simulink model "Servo_Simulation"  (R2019b)
settings: Solver=VariableStepAuto  StartTime=0.0  StopTime=15.0  RelTol=1e-3
undefined symbols (not defined in the file): sigbuilder_block
libraries: simulink x4
settings Model: PacingRate=0.008900  Creator=michi  LastModifiedBy=michi

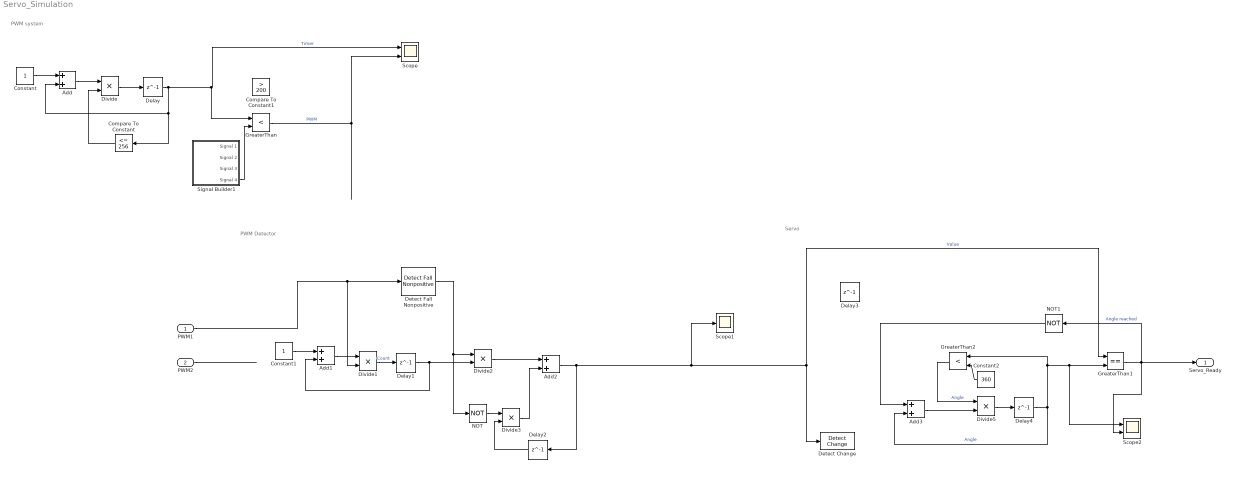
== system Servo_Simulation ==
  note: Servo
  note: PWM Detector
  note: PWM system
  PWM1 : Inport
  PWM2 : Inport  Port=2
  Add{,1..3} (4 alike) : Sum
  Compare To Constant : simulink/Logic and Bit Operations/Compare To Constant  relop=<=  const=256  OutDataTypeStr=boolean
  Compare To Constant1 : simulink/Logic and Bit Operations/Compare To Constant  relop=>  const=200  OutDataTypeStr=boolean
  Constant : Constant
  Constant1 : Constant
  Constant2 : Constant  Value=360
  Delay{,1..3} (4 alike) : Delay  DelayLength=1  SampleTime=1/12800
  Delay4 : Delay  DelayLength=1  SampleTime=0.16/60
  Detect Change : simulink/Logic and Bit Operations/Detect Change  vinit=0  OutDataTypeStr=boolean
  Detect Fall Nonpositive : simulink/Logic and Bit Operations/Detect Fall Nonpositive  vinit=1  OutDataTypeStr=boolean
      settings: SourceProductName=Simulink  SourceProductBaseCode=SL
  Divide : Product  Inputs=**  SaturateOnIntegerOverflow=on  RndMeth=Zero
  Divide1 : Product  Inputs=**  SaturateOnIntegerOverflow=on  RndMeth=Zero
  Divide2 : Product  Inputs=**
  Divide3 : Product  Inputs=**
  Divide5 : Product  Inputs=**  OutDataTypeStr=uint16  SaturateOnIntegerOverflow=on  RndMeth=Zero
  GreaterThan : RelationalOperator  Operator=<  OutDataTypeStr=boolean  RndMeth=Simplest
  GreaterThan1 : RelationalOperator  Operator===  OutDataTypeStr=boolean  RndMeth=Simplest
  GreaterThan2 : RelationalOperator  Operator=<  OutDataTypeStr=boolean  RndMeth=Simplest
  NOT : Logic  Operator=NOT  IconShape=distinctive  AllPortsSameDT=off  OutDataTypeStr=boolean
  NOT1 : Logic  Operator=NOT  IconShape=distinctive  AllPortsSameDT=off  OutDataTypeStr=boolean
  Scope : Scope  NumInputPorts=2
  Scope1 : Scope
  Scope2 : Scope  NumInputPorts=2
  Signal Builder1 : Subsystem  Tag=STV Subsys  LoadFcn=sigbuilder_block('load');  StartFcn=sigbuilder_block('start');  StopFcn=sigbuilder_block('stop');  ClipboardFcn=sigbuilder_block('clipboard');  mask(Sigbuilder block){tuvar=[0:10]}
      mask help: Simulink:masks:SigbuilderBlock_MD
      mask init:
      | if ~strcmp(get_param(bdroot(gcbh),'SimulationStatus'),'stopped') tuvar = sigbuilder_block('maskInit'); end
      settings: CopyFcn=sigbuilder_block('copy');  DeleteFcn=sigbuilder_block('delete');  ModelCloseFcn=sigbuilder_block('modelClose');  PreSaveFcn=sigbuilder_block('preSave');  PauseFcn=sigbuilder_block('pause');  ContinueFcn=sigbuilder_block('continue');  NameChangeFcn=sigbuilder_block('namechange');  OpenFcn=sigbuilder_block('open',[5.5 30 1909 958 ]);  CloseFcn=sigbuilder_block('close');
      mask Display: plot(0, 0, 100, 100,[2, 2, 32, 32, 2], [68, 8, 8, 68, 68],[32, 2], [38, 38], [32, 19, 2],[53, 60, 44], [32, 17, 17, 2],[16, 16, 31, 31]);txt = getActiveGroup(gcbh);text(2, 100, txt,'verticalAlignment', 'top');
  Servo_Ready : Outport
  wires:
  Compare To Constant/1 -> Divide/2
  GreaterThan/1 -> Scope/2  "PWM"
  Add/1 -> Divide/1
  Divide/1 -> Delay/1
  Delay/1 -> GreaterThan/1, Scope/1, Add/2, Compare To Constant/1  "Timer"
  Constant/1 -> Add/1
  Constant1/1 -> Add1/1
  Add1/1 -> Divide1/1
  Divide1/1 -> Delay1/1  "Count"
  Delay1/1 -> Divide2/2, Add1/2
  Detect Fall Nonpositive/1 -> NOT/1, Divide2/1
  Divide2/1 -> Add2/1
  Add2/1 -> GreaterThan1/1, Detect Change/1, Scope1/1, Delay2/1  "Value"
  Delay2/1 -> Divide3/2
  NOT/1 -> Divide3/1
  Divide3/1 -> Add2/2
  Signal Builder1/4(Signal 4) -> GreaterThan/2
  PWM1/1 -> Divide1/2, Detect Fall Nonpositive/1
  PWM2/1 -> ?
  Delay4/1 -> GreaterThan2/1, Scope2/1, GreaterThan1/2, Add3/2  "Angle"
  GreaterThan1/1 -> Scope2/2, NOT1/1, Servo_Ready/1  "Angle reached"
  Add3/1 -> Divide5/2
  NOT1/1 -> Add3/1
  Divide5/1 -> Delay4/1
  Constant2/1 -> GreaterThan2/2
  GreaterThan2/1 -> Divide5/1  "Angle"

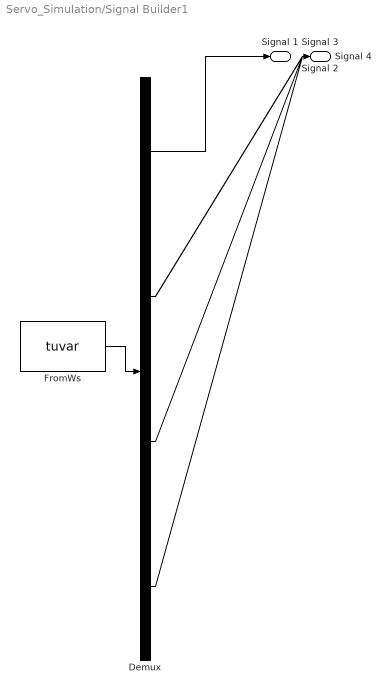
== system Servo_Simulation/Signal Builder1 ==
  Demux : Demux  Tag=STV Demux
  FromWs : FromWorkspace  Tag=STV FromWs  VariableName=tuvar  SampleTime=0
      SigBuilderData=|
      | common.afterFinalStr = 'Extrapolate'
      | common.sampleTime = 0
      | dataSet.timeRange = [0 10]
      | dataSet.name = 'Group 1'
      | sbobj.Groups.Name = 'Group 1'
      | sbobj.Groups.Signals(1).Name = 'Signal 1'
      | sbobj.Groups.Signals(1).XData = [0 4 5 6 10]
      | sbobj.Groups.Signals(1).YData = [0 180 90 90 0]
      | sbobj.Groups.Signals(2).Name = 'Signal 2'
      | sbobj.Groups.Signals(2).XData = [0 2 5 10]
      | sbobj.Groups.Signals(2).YData = [0 0 180 180]
      | sbobj.Groups.Signals(3).Name = 'Signal 3'
      | sbobj.Groups.Signals(3).XData = [0 4 9 10]
      | sbobj.Groups.Signals(3).YData = [0 90 90 0]
      | sbobj.Groups.Signals(4).Name = 'Signal 4'
      | sbobj.Groups.Signals(4).XData = [0 4 4 6 6 10]
      | sbobj.Groups.Signals(4).YData = [0 0 130 130 40 40]
  Signal 1 : Outport  Tag=STV Outport
  Signal 2 : Outport  Tag=STV Outport  Port=2
  Signal 3 : Outport  Tag=STV Outport  Port=3
  Signal 4 : Outport  Tag=STV Outport  Port=4
  wires:
  Demux/1 -> Signal 1/1
  FromWs/1 -> Demux/1
  Demux/2 -> Signal 2/1
  Demux/3 -> Signal 3/1
  Demux/4 -> Signal 4/1
